simulink model "opampschmitttrigger"  (R2026a)
settings: Solver=ode1  StopTime=inf  FixedStep=0.001
undefined symbols (not defined in the file or in its folder): Blocking, Non
libraries: amg_usbconverter_n_connect_lib x2, nesl_utility x1
settings Model: Creator=pboon  LastModifiedBy=Lenovo LOQ

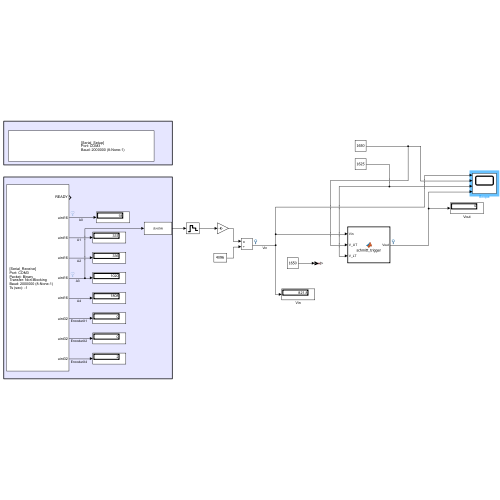
[thumbnail: Simulink's stored preview of the top-level diagram]
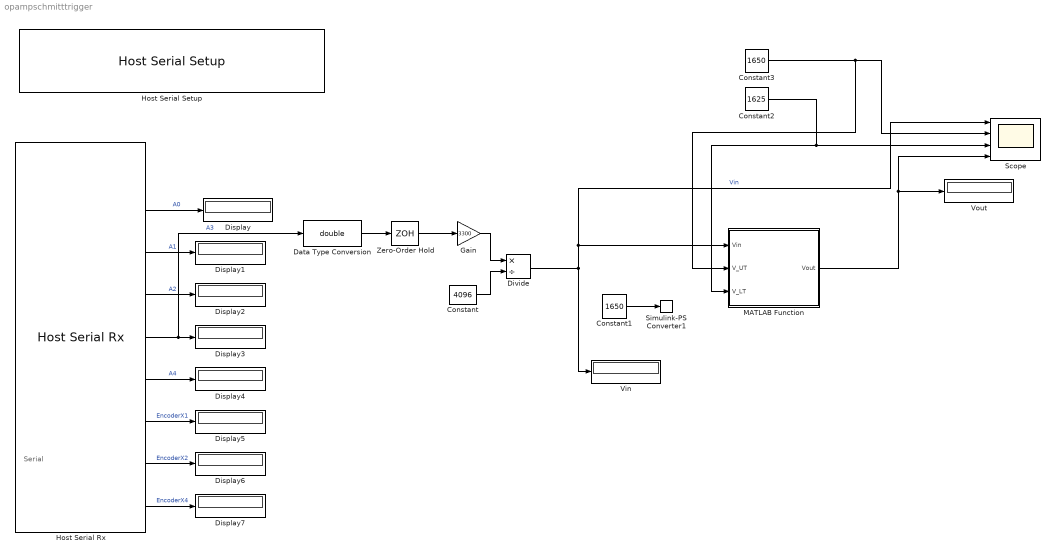
== system opampschmitttrigger ==
  note: Serial
  Constant : Constant  Value=4096
  Constant1 : Constant  Value=1650
  Constant2 : Constant  Value=1625
  Constant3 : Constant  Value=1650
  Data Type Conversion : DataTypeConversion  OutDataTypeStr=double  SaturateOnIntegerOverflow=off  RndMeth=Floor
  Display{,1..7} (8 alike) : Display
  Divide : Product  Inputs=*/
  Gain : Gain  Gain=3300
  Host Serial Rx : amg_usbconverter_n_connect_lib/Host Serial Rx  conf=rx  port=COM3  baudrate=2000000  databits=8  parity=None  stopbit=1  flowcontrol=None  transfer=Non-Blocking  timeout=5  packetmode=Binary  enableinitialvalues=off  initialvalues=[]  binheader='25'  binterminator='4E 4E'  porttype_double=0  porttype_single=0  porttype_int8=0  porttype_uint8=0  porttype_int16=0  porttype_uint16=5  porttype_int32=0  porttype_uint32=3  asciiformat='%d,%f'  rx_asciiterminator="CRLF (0x0D 0x0A - \"\\r\\n\")"  tx_asciiterminator="CRLF (0x0D 0x0A - \"\\r\\n\")"  sampletime=0.001  enablecustomportlabel=off  cinputportlabel=0  coutputportlabel=A  portpinstr=0  blockid=HostSerialRx  inputporttype=[]  inputportwidth=[]  inputportlabel={}  outputporttype=[3 5 5 5 5 5 7 7 7]  outputportwidth=[1 1 1 1 1 1 1 1 1]  outputportlabel={'READY','uint16','uint16','uint16','uint16','uint16','uint32','uint32','uint32'}  compat=0  optionstring=[]  autoport='COM3'
  Host Serial Setup : amg_usbconverter_n_connect_lib/Host Serial Setup  conf=setup  port=COM3  baudrate=2000000  databits=8  parity=None  stopbit=1  flowcontrol=None  transfer=Blocking  timeout=2  packetmode=Binary  initialvalues=[]  binheader='7E 7E'  binterminator='03 03'  porttype_double=0  porttype_single=1  porttype_int8=0  porttype_uint8=0  porttype_int16=0  porttype_uint16=0  porttype_int32=0  porttype_uint32=2  asciiformat='%d %u %x'  rx_asciiterminator="CRLF (0x0D 0x0A - \"\\r\\n\")"  tx_asciiterminator="CRLF (0x0D 0x0A - \"\\r\\n\")"  sampletime=-1  enablecustomportlabel=off  cinputportlabel=0  coutputportlabel=A  portpinstr=0  blockid=HostSerialSetup  inputporttype=[]  inputportwidth=[]  inputportlabel={}  outputporttype=[]  outputportwidth=[]  outputportlabel={}  compat=0  optionstring=[]  autoport='COM3'
  MATLAB Function : MATLAB Function  TreatAsAtomicUnit=on
  Scope : Scope  NumInputPorts=4
      settings: ActiveDisplayYMinimum=-334.95483398437494  ActiveDisplayYMaximum=3014.593505859375
  Simulink-PS Converter1 : nesl_utility/Simulink-PS Converter  PhysicalDomain=network_engine_domain  SubClassName=ps_input  LeftPortType=input  RightPortType=output  PseudoPeriodic=off  Frequencies=[]  NoiseDistribution=none  NoiseParameters=[]  Unit=1  AffineConversion=off  FilteringAndDerivatives=provide  SimscapeFilterOrder=1  InputFilterTimeConstant=0.001  UdotUserProvided=0
  Vin : Display
  Vout : Display
  Zero-Order Hold : ZeroOrderHold  SampleTime=0.001
  wires:
  Host Serial Rx/2 -> Display/1  "A0"
  Host Serial Rx/3 -> Display1/1  "A1"
  Host Serial Rx/4 -> Display2/1  "A2"
  Host Serial Rx/5 -> Data Type Conversion/1, Display3/1  "A3"
  Host Serial Rx/6 -> Display4/1  "A4"
  Host Serial Rx/7 -> Display5/1  "EncoderX1"
  Host Serial Rx/8 -> Display6/1  "EncoderX2"
  Host Serial Rx/9 -> Display7/1  "EncoderX4"
  Gain/1 -> Divide/1
  Constant/1 -> Divide/2
  Divide/1 -> MATLAB Function/1(Vin), Scope/1, Vin/1  "Vin"
  Zero-Order Hold/1 -> Gain/1
  Data Type Conversion/1 -> Zero-Order Hold/1
  Constant1/1 -> Simulink-PS Converter1/1
  MATLAB Function/1(Vout) -> Scope/4, Vout/1
  Constant3/1 -> Scope/2, MATLAB Function/2(V_UT)
  Constant2/1 -> Scope/3, MATLAB Function/3(V_LT)

== matlab function opampschmitttrigger/MATLAB Function ==
  data: Vin input; Vout output; V_UT input; V_LT input
function Vout = schmitt_trigger(Vin, V_UT, V_LT)

    persistent Vout_prev;

    if isempty(Vout_prev)
        Vout_prev = 0; % เริ่มต้นสถานะ LOW (0)
    end
    
    if Vin > V_UT
        Vout = 1000;      % สวิตช์เป็น HIGH (1000) เมื่ออินพุตสูงข้าม V_UT
    elseif Vin < V_LT
        Vout = 0;         % สวิตช์เป็น LOW (0) เมื่ออินพุตลดลงต่ำกว่า V_LT
    else
        Vout = Vout_prev; % อยู่ในช่วง Hysteresis ให้คงสถานะเดิมไว้
    end
  
    Vout_prev = Vout;
end
